simulink model "OBSTACLEDETECTOR"  (R2023b)
settings: Solver=VariableStepAuto  StartTime=0.0  StopTime=10.0  RelTol=1e-3
settings Model: Creator=lucaerviati  LastModifiedBy=monis
settings OptimizationCC: ReuseModelBlockBuffer=off

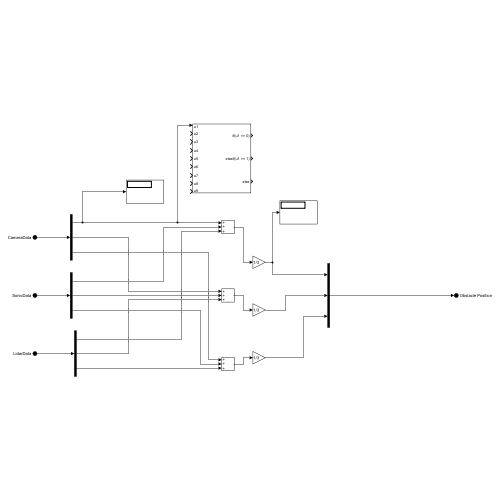
[thumbnail: Simulink's stored preview of the top-level diagram]
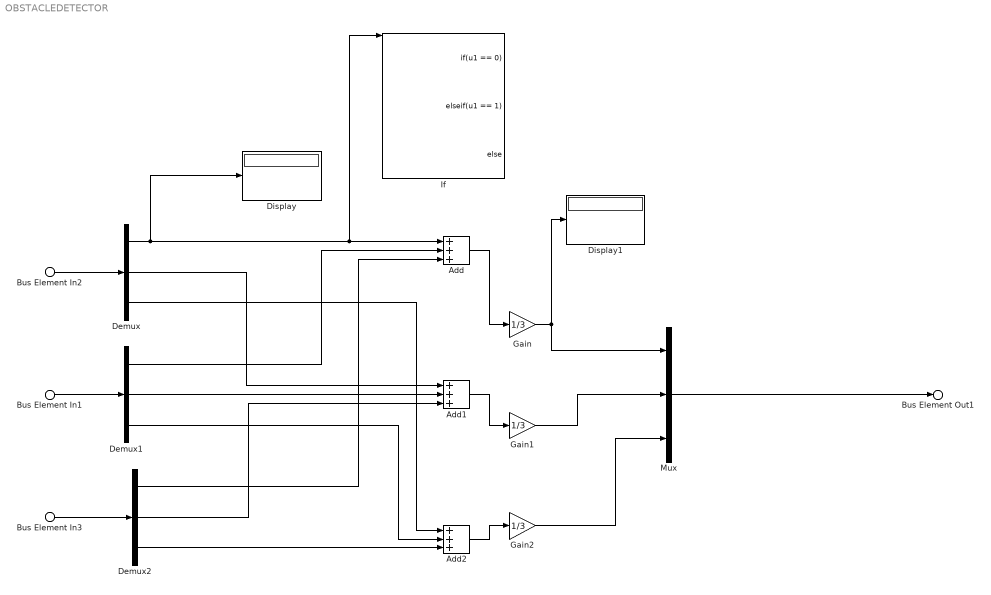
== system OBSTACLEDETECTOR ==
  Bus Element In2 : Inport  PortName=CameraData
  Bus Element In1 : Inport  Port=2  PortName=SonicData
  Bus Element In3 : Inport  Port=3  PortName=LidarData
  Add : Sum  Inputs=+++
  Add1 : Sum  Inputs=+++
  Add2 : Sum  Inputs=+++
  Demux : Demux  Outputs=3
  Demux1 : Demux  Outputs=3
  Demux2 : Demux  Outputs=3
  Display : Display
  Display1 : Display
  Gain : Gain  Gain=1/3
  Gain1 : Gain  Gain=1/3
  Gain2 : Gain  Gain=1/3
  If : If  NumInputs=9  IfExpression=u1 == 0  ElseIfExpressions=u1 == 1
  Mux : Mux  Inputs=3
  Bus Element Out1 : Outport  PortName=Obstacle Position
  wires:
  Bus Element In2/1 -> Demux/1
  Bus Element In1/1 -> Demux1/1
  Bus Element In3/1 -> Demux2/1
  Demux/1 -> If/1, Add/1, Display/1
  Demux1/1 -> Add/2
  Demux2/1 -> Add/3
  Add/1 -> Gain/1
  Gain/1 -> Mux/1, Display1/1
  Add2/1 -> Gain2/1
  Add1/1 -> Gain1/1
  Demux/2 -> Add1/1
  Demux1/2 -> Add1/2
  Demux2/2 -> Add1/3
  Demux/3 -> Add2/1
  Demux1/3 -> Add2/2
  Demux2/3 -> Add2/3
  Gain1/1 -> Mux/2
  Gain2/1 -> Mux/3
  Mux/1 -> Bus Element Out1/1
